simulink model "DR_Screening_Capacity_Model"  (R2024b)
settings: Solver=FixedStepDiscrete  StartTime=0.0  StopTime=cfg.campDurationSeconds  RelTol=1e-3
values from neighbouring files (symbols this model uses):
  cfg = struct()    [config.m]
  m = simulate_capacity_scenario(cfgRun)    [run_resource_optimization.m]
  n = height(measurements)    [generate_telemetry.m]
settings Model: Creator=Chait  LastModifiedBy=Chait

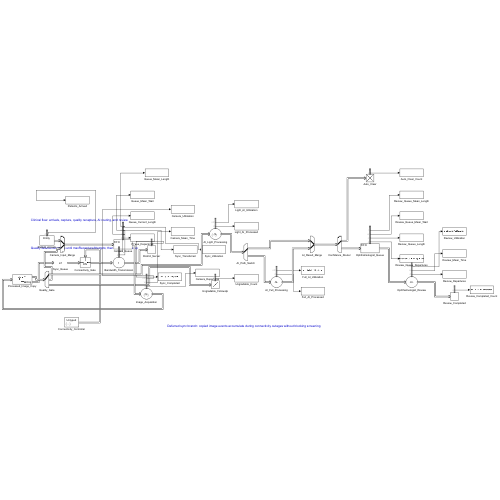
[thumbnail: Simulink's stored preview of the top-level diagram]
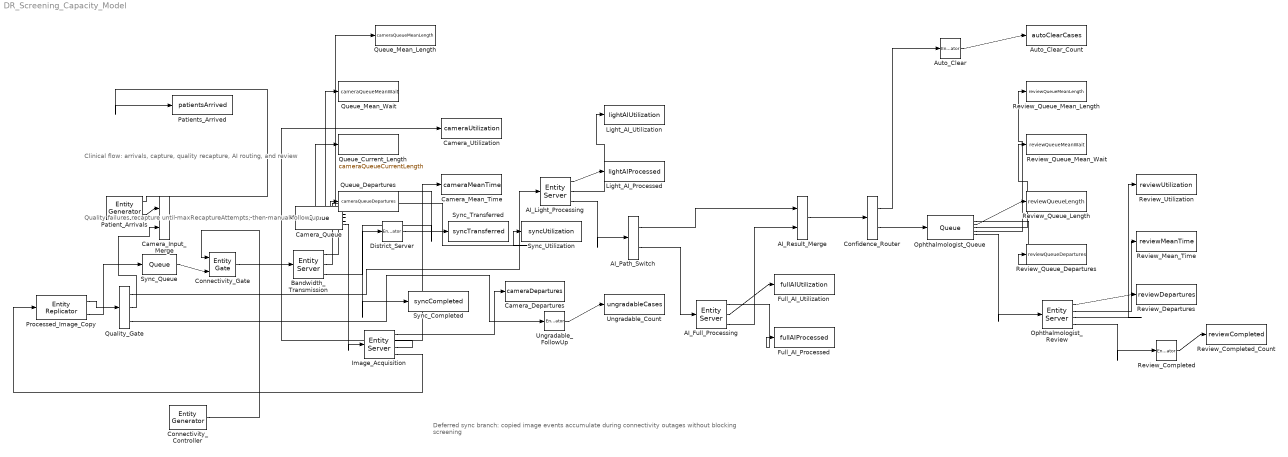
== system DR_Screening_Capacity_Model ==
  note: Clinical flow: arrivals, capture, quality recapture, AI routing, and review
  note: Quality failures recapture until maxRecaptureAttempts; then manual follow-up
  note: Deferred sync branch: copied image events accumulate during connectivity outages without blocking screening
  AI_Full_Processing : EntityServer  InputPortMessageModes=m  OutputPortMessageModes=n,n,m  Capacity=cfg.numAIDevices  ServiceTimeValue=cfg.fullPathLatency  NumberEntitiesDeparted=on  Utilization=on
      settings: OutputPortMap=o0,o5,o9
  AI_Light_Processing : EntityServer  InputPortMessageModes=m  OutputPortMessageModes=n,n,m  Capacity=cfg.numAIDevices  ServiceTimeValue=cfg.lightPathLatency  ServiceCompleteAction=coder.extrinsic('rand'); pathDraw = 1; pathDraw = rand(); entity.AIPath = 1; if pathDraw < cfg.fullPathProbability, entity.AIPath = 2; end; confidenceDraw = 1; confidenceDraw = rand(); entity.ReviewRoute = 2; if confidenceDraw >= cfg.confidenceThreshold, entity.ReviewRoute = 1; end;  NumberEntitiesDeparted=on  Utilization=on
      settings: OutputPortMap=o0,o5,o9
  AI_Path_Switch : EntityOutputSwitch  InputPortMessageModes=m  OutputPortMessageModes=m,m  SwitchingCriterion=From attribute  SwitchAttributeName=AIPath
  AI_Result_Merge : EntityInputSwitch  InputPortMessageModes=m,m  OutputPortMessageModes=m
  Auto_Clear : EntityTerminator  InputPortMessageModes=m  NumberEntitiesArrived=on
      settings: OutputPortMap=o0
  Auto_Clear_Count : ToWorkspace  VariableName=autoClearCases  SaveFormat=Timeseries  SampleTime=-1
  Bandwidth_Transmission : EntityServer  InputPortMessageModes=m  OutputPortMessageModes=n,n,m  Capacity=1  ServiceTimeValue=cfg.imageSizeMB*8/cfg.bandwidthMbps  NumberEntitiesDeparted=on  Utilization=on
      settings: OutputPortMap=o0,o5,o9
  Camera_Departures : ToWorkspace  VariableName=cameraDepartures  SaveFormat=Timeseries  SampleTime=-1
  Camera_Input_Merge : EntityInputSwitch  InputPortMessageModes=m,m  OutputPortMessageModes=m
  Camera_Mean_Time : ToWorkspace  VariableName=cameraMeanTime  SaveFormat=Timeseries  SampleTime=-1
  Camera_Queue : Queue  InputPortMessageModes=m  OutputPortMessageModes=n,n,n,n,m  Capacity=cfg.cameraQueueCapacity  NumberEntitiesDeparted=on  NumberEntitiesInBlock=on  AverageWait=on  AverageQueueLength=on
      settings: OutputPortMap=o0,o1,o2,o3,o5
  Camera_Utilization : ToWorkspace  VariableName=cameraUtilization  SaveFormat=Timeseries  SampleTime=-1
  Confidence_Router : EntityOutputSwitch  InputPortMessageModes=m  OutputPortMessageModes=m,m  SwitchingCriterion=From attribute  SwitchAttributeName=ReviewRoute
  Connectivity_Controller : EntityGenerator  OutputPortMessageModes=m  TimeSource=MATLAB action  IntergenerationTimeAction=persistent eventIndex; if isempty(eventIndex), eventIndex = 1; end; dt = cfg.syncEventIntervals(eventIndex); eventIndex = mod(eventIndex,numel(cfg.syncEventIntervals)) + 1;  GenerateEntityAtSimulationStart=off  GenerateAction=persistent isOnline; if isempty(isOnline), isOnline = 1; else, isOnline = 1 - isOnline; end; entity = isOnline;  EntityTypeName=Entity
  Connectivity_Gate : EntityGate  InputPortMessageModes=m,m  OutputPortMessageModes=m
  District_Server : EntityTerminator  InputPortMessageModes=m  NumberEntitiesArrived=on
      settings: OutputPortMap=o0
  Full_AI_Processed : ToWorkspace  VariableName=fullAIProcessed  SaveFormat=Timeseries  SampleTime=-1
  Full_AI_Utilization : ToWorkspace  VariableName=fullAIUtilization  SaveFormat=Timeseries  SampleTime=-1
  Image_Acquisition : EntityServer  InputPortMessageModes=m  OutputPortMessageModes=n,n,n,m  Capacity=cfg.numCameras  ServiceTimeValue=cfg.acquisitionTime  ServiceCompleteAction=coder.extrinsic('rand'); qualityDraw = 1; qualityDraw = rand(); if qualityDraw < cfg.qualityRejectRate, entity.RecaptureAttempts = entity.RecaptureAttempts + 1; if entity.RecaptureAttempts > cfg.maxRecaptureAttempts, entity.QualityRoute = 3; else, entity.QualityRoute = 2; end; else, entity.QualityRoute = 1; end;  NumberEntitiesDeparted=on  AverageWait=on  Utilization=on
      settings: OutputPortMap=o0,o4,o5,o9
  Light_AI_Processed : ToWorkspace  VariableName=lightAIProcessed  SaveFormat=Timeseries  SampleTime=-1
  Light_AI_Utilization : ToWorkspace  VariableName=lightAIUtilization  SaveFormat=Timeseries  SampleTime=-1
  Ophthalmologist_Queue : Queue  InputPortMessageModes=m  OutputPortMessageModes=n,n,n,n,m  Capacity=inf  NumberEntitiesDeparted=on  NumberEntitiesInBlock=on  AverageWait=on  AverageQueueLength=on
      settings: OutputPortMap=o0,o1,o2,o3,o5
  Ophthalmologist_Review : EntityServer  InputPortMessageModes=m  OutputPortMessageModes=n,n,n,m  Capacity=cfg.numOphthalmologists  ServiceTimeValue=cfg.reviewTime  NumberEntitiesDeparted=on  AverageWait=on  Utilization=on
      settings: OutputPortMap=o0,o4,o5,o9
  Patient_Arrivals : EntityGenerator  OutputPortMessageModes=n,m  Period=cfg.meanInterarrivalTime  IntergenerationTimeAction=dt = cfg.meanInterarrivalTime;  AttributeName=QualityRoute|RecaptureAttempts|AIPath|ReviewRoute  AttributeInitialValue=1|0|1|1  NumberEntitiesDeparted=on  EntityType=Structured  EntityTypeName=Entity
      settings: OutputPortMap=o0,o3
  Patients_Arrived : ToWorkspace  VariableName=patientsArrived  SaveFormat=Timeseries  SampleTime=-1
  Processed_Image_Copy : EntityReplicator  InputPortMessageModes=m  OutputPortMessageModes=m,m
  Quality_Gate : EntityOutputSwitch  InputPortMessageModes=m  OutputPortMessageModes=m,m,m  NumberOutputPorts=3  SwitchingCriterion=From attribute  SwitchAttributeName=QualityRoute
      settings: OutputPortMap=o0,o1,o2
  Queue_Current_Length : ToWorkspace  VariableName=cameraQueueCurrentLength  SaveFormat=Timeseries  SampleTime=-1
  Queue_Departures : ToWorkspace  VariableName=cameraQueueDepartures  SaveFormat=Timeseries  SampleTime=-1
  Queue_Mean_Length : ToWorkspace  VariableName=cameraQueueMeanLength  SaveFormat=Timeseries  SampleTime=-1
  Queue_Mean_Wait : ToWorkspace  VariableName=cameraQueueMeanWait  SaveFormat=Timeseries  SampleTime=-1
  Review_Completed : EntityTerminator  InputPortMessageModes=m  NumberEntitiesArrived=on
      settings: OutputPortMap=o0
  Review_Completed_Count : ToWorkspace  VariableName=reviewCompleted  SaveFormat=Timeseries  SampleTime=-1
  Review_Departures : ToWorkspace  VariableName=reviewDepartures  SaveFormat=Timeseries  SampleTime=-1
  Review_Mean_Time : ToWorkspace  VariableName=reviewMeanTime  SaveFormat=Timeseries  SampleTime=-1
  Review_Queue_Departures : ToWorkspace  VariableName=reviewQueueDepartures  SaveFormat=Timeseries  SampleTime=-1
  Review_Queue_Length : ToWorkspace  VariableName=reviewQueueLength  SaveFormat=Timeseries  SampleTime=-1
  Review_Queue_Mean_Length : ToWorkspace  VariableName=reviewQueueMeanLength  SaveFormat=Timeseries  SampleTime=-1
  Review_Queue_Mean_Wait : ToWorkspace  VariableName=reviewQueueMeanWait  SaveFormat=Timeseries  SampleTime=-1
  Review_Utilization : ToWorkspace  VariableName=reviewUtilization  SaveFormat=Timeseries  SampleTime=-1
  Sync_Completed : ToWorkspace  VariableName=syncCompleted  SaveFormat=Timeseries  SampleTime=-1
  Sync_Queue : Queue  InputPortMessageModes=m  OutputPortMessageModes=m  OverwriteOldest=on  Capacity=inf  NumberEntitiesDeparted=on  NumberEntitiesInBlock=on  AverageWait=on  AverageQueueLength=on
  Sync_Transferred : ToWorkspace  VariableName=syncTransferred  SaveFormat=Timeseries  SampleTime=-1
  Sync_Utilization : ToWorkspace  VariableName=syncUtilization  SaveFormat=Timeseries  SampleTime=-1
  Ungradable_Count : ToWorkspace  VariableName=ungradableCases  SaveFormat=Timeseries  SampleTime=-1
  Ungradable_FollowUp : EntityTerminator  InputPortMessageModes=m  NumberEntitiesArrived=on
      settings: OutputPortMap=o0
  wires:
  Ophthalmologist_Queue/1 -> Review_Queue_Departures/1
  AI_Full_Processing/2 -> Full_AI_Utilization/1
  AI_Full_Processing/1 -> Full_AI_Processed/1
  AI_Light_Processing/2 -> Light_AI_Utilization/1
  AI_Light_Processing/1 -> Light_AI_Processed/1
  Ungradable_FollowUp/1 -> Ungradable_Count/1
  AI_Light_Processing/3 -> AI_Path_Switch/1
  AI_Path_Switch/1 -> AI_Result_Merge/1
  AI_Path_Switch/2 -> AI_Full_Processing/1
  AI_Full_Processing/3 -> AI_Result_Merge/2
  AI_Result_Merge/1 -> Confidence_Router/1
  Confidence_Router/1 -> Auto_Clear/1
  Auto_Clear/1 -> Auto_Clear_Count/1
  Confidence_Router/2 -> Ophthalmologist_Queue/1
  Ophthalmologist_Queue/5 -> Ophthalmologist_Review/1
  Ophthalmologist_Review/4 -> Review_Completed/1
  Ophthalmologist_Queue/2 -> Review_Queue_Length/1
  Ophthalmologist_Queue/3 -> Review_Queue_Mean_Wait/1
  Ophthalmologist_Queue/4 -> Review_Queue_Mean_Length/1
  Ophthalmologist_Review/1 -> Review_Departures/1
  Ophthalmologist_Review/2 -> Review_Mean_Time/1
  Ophthalmologist_Review/3 -> Review_Utilization/1
  Review_Completed/1 -> Review_Completed_Count/1
  Sync_Queue/1 -> Connectivity_Gate/2
  Connectivity_Controller/1 -> Connectivity_Gate/1
  Bandwidth_Transmission/1 -> Sync_Transferred/1
  Bandwidth_Transmission/2 -> Sync_Utilization/1
  District_Server/1 -> Sync_Completed/1
  Processed_Image_Copy/2 -> Sync_Queue/1
  Connectivity_Gate/1 -> Bandwidth_Transmission/1
  Bandwidth_Transmission/3 -> District_Server/1
  Patient_Arrivals/2 -> Camera_Input_Merge/1
  Camera_Input_Merge/1 -> Camera_Queue/1
  Quality_Gate/2 -> Camera_Input_Merge/2
  Quality_Gate/3 -> Ungradable_FollowUp/1
  Quality_Gate/1 -> AI_Light_Processing/1
  Image_Acquisition/4 -> Processed_Image_Copy/1
  Processed_Image_Copy/1 -> Quality_Gate/1
  Camera_Queue/5 -> Image_Acquisition/1
  Camera_Queue/1 -> Queue_Departures/1
  Camera_Queue/2 -> Queue_Current_Length/1
  Camera_Queue/3 -> Queue_Mean_Wait/1
  Camera_Queue/4 -> Queue_Mean_Length/1
  Image_Acquisition/1 -> Camera_Departures/1
  Image_Acquisition/3 -> Camera_Utilization/1
  Image_Acquisition/2 -> Camera_Mean_Time/1
  Patient_Arrivals/1 -> Patients_Arrived/1
